simulink model "openloop"  (R2021b)
settings: Solver=ode15s  StartTime=0.0  StopTime=50  FixedStep=0.01  RelTol=1e-5  AbsTol=1e-8
values from neighbouring files (symbols this model uses):
  carb1 = 0    [olasm1init.m]
  carb2 = 0    [olasm1init.m]
  carb3 = 0    [olasm1init.m]
  carb4 = 0    [olasm1init.m]
  carb5 = 0    [olasm1init.m]
  DIM = [ area height ]    [olsettler1dinit.m]
  KLa1 = 0    [olasm1init.m]
  KLa2 = 0    [olasm1init.m]
  KLa3 = 240    [olasm1init.m]
  KLa4 = 240    [olasm1init.m]
  KLa5 = 84    [olasm1init.m]
  LAYER = [ feedlayer nooflayers ]    [olsettler1dinit.m]
  MODELTYPE = [ 0 ]    [olsettler1dinit.m]
  PAR1 = [ mu_H  K_S  K_OH  K_NO  b_H  mu_A  K_NH  K_OA  b_A  ny_g  k_a  k_h  K_X  ny_h  Y_H  Y_A  f_P  i_XB  i_XP X_I2TSS  X_S2TSS  X_BH2TSS  X_BA2TSS  X_P2TSS ]    [olasm1init.m]
  PAR2 = PAR1    [olasm1init.m]
  PAR3 = PAR1    [olasm1init.m]
  PAR4 = PAR1    [olasm1init.m]
  PAR5 = PAR1    [olasm1init.m]
  Qin0 = 18446    [olasm1init.m]    (also in statesetol.m)
  Qintr = 3*Qin0    (= 55338)    [olasm1init.m]    (also in statesetol.m)
  SETTLERINIT = [ TSS_1 TSS_2 TSS_3 TSS_4 TSS_5 TSS_6 TSS_7 TSS_8 TSS_9 TSS_10  SI_1 SI_2 SI_3 SI_4 SI_5 SI_6 SI_7 SI_8 SI_9 SI_10  SS_1 SS_2 SS_3 SS_4 SS_5 SS_6 SS_7 SS_8 SS_9 SS_10  SO_1 SO_2 SO_3 SO_4 SO_5 SO_6 SO_7 SO_8 SO_9 SO_10  SNO_1 SNO_2 SNO_3 SNO_4 SNO_5 SNO_6 SNO_7 SNO_8 SNO_9 SNO_10  SNH_1 SNH_2 SNH_3 SNH_4 SNH_5 SNH_6 SNH_7 SNH_8 SNH_9 SNH_10 SND_1 SND_2 SND_3 SND_4 SND_5 SND_6 SND_7 SND_8 SND_9 SND ...(+77 chars)    [olsettler1dinit.m]    (also in savestates.m; savestatesdyn.m; statesetol.m)
  SETTLERPAR = [ v0_max v0 r_h r_p f_ns X_t ]    [olsettler1dinit.m]
  SOSAT1 = 8    [olasm1init.m]
  SOSAT2 = SOSAT1    (= 8)    [olasm1init.m]
  SOSAT3 = SOSAT1    (= 8)    [olasm1init.m]
  SOSAT4 = SOSAT1    (= 8)    [olasm1init.m]
  SOSAT5 = SOSAT1    (= 8)    [olasm1init.m]
  T = 0.0002    [olasm1init.m]
  VOL1 = 1000    [olasm1init.m]
  VOL2 = VOL1    (= 1000)    [olasm1init.m]
  VOL3 = 1333    [olasm1init.m]
  VOL4 = VOL3    (= 1333)    [olasm1init.m]
  VOL5 = VOL3    (= 1333)    [olasm1init.m]
  XINIT1 = XINIT1.*(rand(1, 15)/2)    [olasm1init.m]    (also in savestates.m = [ S_I1  S_S1  X_I1  X_S1  X_BH1  X_BA1  X_P1  S_O1  S_NO1  S; savestatesdyn.m = [ S_I1  S_S1  X_I1  X_S1  X_BH1  X_BA1  X_P1  S_O1  S_NO1  S; statesetol.m = [ S_I1  S_S1  X_I1  X_S1  X_BH1  X_BA1  X_P1  S_O1  S_NO1  S)
  XINIT2 = XINIT2.*(rand(1, 15)/2)    [olasm1init.m]    (also in savestates.m = [ S_I2  S_S2  X_I2  X_S2  X_BH2  X_BA2  X_P2  S_O2  S_NO2  S; savestatesdyn.m = [ S_I2  S_S2  X_I2  X_S2  X_BH2  X_BA2  X_P2  S_O2  S_NO2  S; statesetol.m = [ S_I2  S_S2  X_I2  X_S2  X_BH2  X_BA2  X_P2  S_O2  S_NO2  S)
  XINIT3 = XINIT3.*(rand(1, 15)/2)    [olasm1init.m]    (also in savestates.m = [ S_I3  S_S3  X_I3  X_S3  X_BH3  X_BA3  X_P3  S_O3  S_NO3  S; savestatesdyn.m = [ S_I3  S_S3  X_I3  X_S3  X_BH3  X_BA3  X_P3  S_O3  S_NO3  S; statesetol.m = [ S_I3  S_S3  X_I3  X_S3  X_BH3  X_BA3  X_P3  S_O3  S_NO3  S)
  XINIT4 = XINIT4.*(rand(1, 15)/2)    [olasm1init.m]    (also in savestates.m = [ S_I4  S_S4  X_I4  X_S4  X_BH4  X_BA4  X_P4  S_O4  S_NO4  S; savestatesdyn.m = [ S_I4  S_S4  X_I4  X_S4  X_BH4  X_BA4  X_P4  S_O4  S_NO4  S; statesetol.m = [ S_I4  S_S4  X_I4  X_S4  X_BH4  X_BA4  X_P4  S_O4  S_NO4  S)
  XINIT5 = XINIT5.*(rand(1, 15)/2)    [olasm1init.m]    (also in savestates.m = [ S_I5  S_S5  X_I5  X_S5  X_BH5  X_BA5  X_P5  S_O5  S_NO5  S; savestatesdyn.m = [ S_I5  S_S5  X_I5  X_S5  X_BH5  X_BA5  X_P5  S_O5  S_NO5  S; statesetol.m = [ S_I5  S_S5  X_I5  X_S5  X_BH5  X_BA5  X_P5  S_O5  S_NO5  S)
  XINITDELAY = [ S_I_ASin  S_S_ASin  X_I_ASin  X_S_ASin  X_BH_ASin  X_BA_ASin  X_P_ASin  S_O_ASin  S_NO_ASin  S_NH_ASin  S_ND_ASin  X_ND_ASin  S_ALK_ASin TSS_ASin Q_ASin ]    [olasm1init.m]    (also in savestates.m; savestatesdyn.m; statesetol.m)
settings Model: Creator=ielulf  LastModifiedBy=Yalin
settings SolverCC: AutoScaleAbsTol=off  AlgebraicLoopSolver=TrustRegion
settings DataIOCC: LimitDataPoints=on  SaveFormat=Array  SignalLoggingSaveFormat=ModelDataLogs  SaveOutput=off  ReturnWorkspaceOutputs=off  TimeSaveName=t  SignalLoggingName=sigsOut  OutputOption=SpecifiedOutputTimes  OutputTimes=[0:1:50]
settings OptimizationCC: BlockReduction=off  BooleanDataType=off  InitFltsAndDblsToZero=on  LifeSpan=inf
settings DebuggingCC: SaveWithParameterizedLinksMsg=none  UnderspecifiedInitializationDetection=Classic  MergeDetectMultiDrivingBlocksExec=none  SignalResolutionControl=TryResolveAllWithWarning  InheritedTsInSrcMsg=none  MultiTaskDSMMsg=warning  MultiTaskCondExecSysMsg=none  FcnCallInpInsideContextMsg=warning  UnconnectedOutputMsg=none  SFUnexpectedBacktrackingDiag=warning  SFNoUnconditionalDefaultTransitionDiag=warning  SFExecutionAtInitializationDiag=none  SFMachineParentedDataDiag=warning  ArithmeticOperatorsInVariantConditions=warning
settings HardwareCC: ProdBitPerPointer=32  ProdBitPerSizeT=32  ProdBitPerPtrDiffT=32  ProdLargestAtomicFloat=None  ProdIntDivRoundTo=Undefined  ProdEndianess=Unspecified  ProdWordSize=32  ProdHWDeviceType=32-bit Generic  TargetUnknown=on
settings ModelReferenceCC: PropagateSignalLabelsOutOfModel=off
settings RTWCC: TemplateMakefile=grt_unix.tmf
settings CodeAppCC: StateflowObjectComments=on
settings GRTTargetCC: TargetFcnLib=ansi_tfl_tmw.mat  TargetLangStandard=C89/C90 (ANSI)  CombineOutputUpdateFcns=off  GRTInterface=on
settings ConfigComp: CovMetricSettings=dw  CovSaveCumulativeToWorkspaceVar=on  CovSaveSingleToWorkspaceVar=on

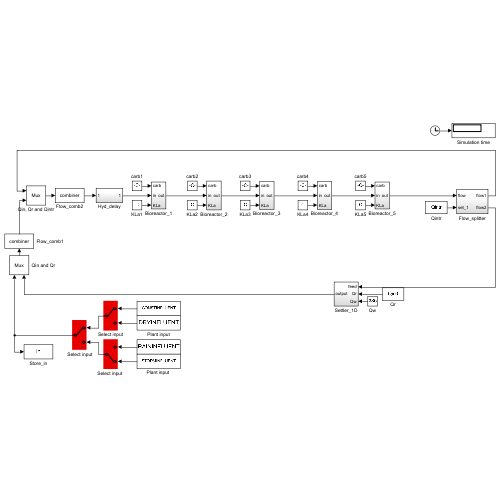
[thumbnail: Simulink's stored preview of the top-level diagram]
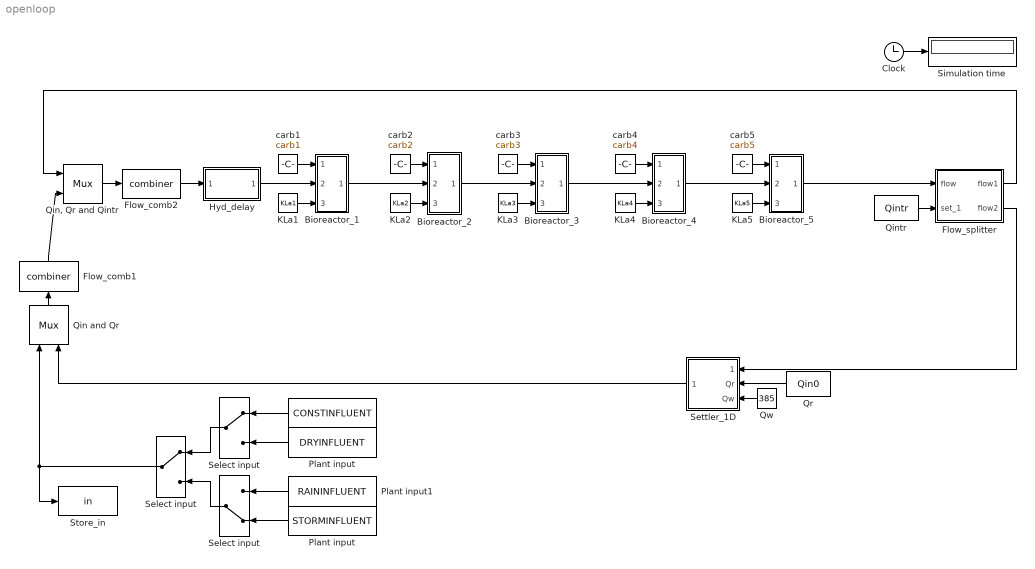
== system openloop ==
  " " : FromWorkspace  VariableName=CONSTINFLUENT  SampleTime=-1  ZeroCross=off  OutputAfterFinalValue=Holding final value
  " Select input" : ManualSwitch
  Bioreactor_1 : Subsystem
  Bioreactor_2 : Subsystem
  Bioreactor_3 : Subsystem
  Bioreactor_4 : Subsystem
  Bioreactor_5 : Subsystem
  Clock : Clock
  Flow_comb1 : S-Function  FunctionName=combiner  SFunctionDeploymentMode=off  EnableBusSupport=off
  Flow_comb2 : S-Function  FunctionName=combiner  SFunctionDeploymentMode=off  EnableBusSupport=off
  Flow_splitter : Subsystem
  Hyd_delay : Subsystem
  KLa1 : Constant  Value=KLa1
  KLa2 : Constant  Value=KLa2
  KLa3 : Constant  Value=KLa3
  KLa4 : Constant  Value=KLa4
  KLa5 : Constant  Value=KLa5
  Plant input : FromWorkspace  VariableName=DRYINFLUENT  SampleTime=-1  ZeroCross=off  OutputAfterFinalValue=Holding final value
  "Plant input " : FromWorkspace  VariableName=STORMINFLUENT  SampleTime=-1  ZeroCross=off  OutputAfterFinalValue=Holding final value
  Plant input1 : FromWorkspace  VariableName=RAININFLUENT  SampleTime=-1  ZeroCross=off  OutputAfterFinalValue=Holding final value
  Qin and Qr : Mux  Inputs=2
  "Qin, Qr and Qintr" : Mux  Inputs=2
  Qintr : Constant  Value=Qintr
  Qr : Constant  Value=Qin0
  Qw : Constant  Value=385
  Select input : ManualSwitch
  "Select input " : ManualSwitch  CurrentSetting=0
  Settler_1D : Subsystem
  Simulation time : Display
  Store_in : ToWorkspace  VariableName=in  SampleTime=-1
  carb1 : Constant  Value=carb1
  carb2 : Constant  Value=carb2
  carb3 : Constant  Value=carb3
  carb4 : Constant  Value=carb4
  carb5 : Constant  Value=carb5
  wires:
  Qin and Qr/1 -> Flow_comb1/1
  Flow_comb1/1 -> "Qin, Qr and Qintr"/2
  "Qin, Qr and Qintr"/1 -> Flow_comb2/1
  Flow_splitter/1(flow1) -> "Qin, Qr and Qintr"/1
  Settler_1D/1(output) -> Qin and Qr/2
  Qw/1 -> Settler_1D/3(Qw)
  Flow_splitter/2(flow2) -> Settler_1D/1(feed)
  Qintr/1 -> Flow_splitter/2(set_1)
  Qr/1 -> Settler_1D/2(Qr)
  Bioreactor_5/1(out) -> Flow_splitter/1(flow)
  Flow_comb2/1 -> Hyd_delay/1(Input)
  Clock/1 -> Simulation time/1
  Plant input/1 -> Select input/2
  " "/1 -> Select input/1
  Hyd_delay/1(Output) -> Bioreactor_1/2(in)
  carb1/1 -> Bioreactor_1/1(carb)
  KLa1/1 -> Bioreactor_1/3(KLa)
  Bioreactor_1/1(out) -> Bioreactor_2/2(in)
  KLa2/1 -> Bioreactor_2/3(KLa)
  carb2/1 -> Bioreactor_2/1(carb)
  Bioreactor_2/1(out) -> Bioreactor_3/2(in)
  KLa3/1 -> Bioreactor_3/3(KLa)
  carb3/1 -> Bioreactor_3/1(carb)
  Bioreactor_3/1(out) -> Bioreactor_4/2(in)
  KLa4/1 -> Bioreactor_4/3(KLa)
  carb4/1 -> Bioreactor_4/1(carb)
  Bioreactor_4/1(out) -> Bioreactor_5/2(in)
  KLa5/1 -> Bioreactor_5/3(KLa)
  carb5/1 -> Bioreactor_5/1(carb)
  Plant input1/1 -> "Select input "/1
  "Plant input "/1 -> "Select input "/2
  Select input/1 -> " Select input"/1
  "Select input "/1 -> " Select input"/2
  " Select input"/1 -> Qin and Qr/1, Store_in/1

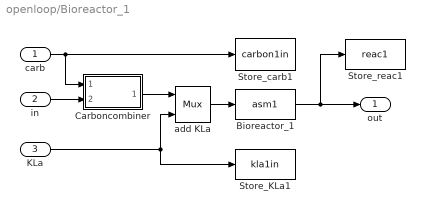
== system openloop/Bioreactor_1 ==
  carb : Inport
  in : Inport  Port=2
  KLa : Inport  Port=3
  Bioreactor_1 : S-Function  FunctionName=asm1  Parameters=XINIT1,PAR1,VOL1,SOSAT1  SFunctionDeploymentMode=off  EnableBusSupport=off
  Carboncombiner : Subsystem
  Store_KLa1 : ToWorkspace  VariableName=kla1in  SampleTime=-1
  Store_carb1 : ToWorkspace  VariableName=carbon1in  SampleTime=-1
  Store_reac1 : ToWorkspace  VariableName=reac1  SampleTime=-1
  add KLa : Mux  Inputs=2
  out : Outport
  wires:
  add KLa/1 -> Bioreactor_1/1
  Bioreactor_1/1 -> out/1, Store_reac1/1
  Carboncombiner/1(Output) -> add KLa/1
  carb/1 -> Store_carb1/1, Carboncombiner/1(C_flow)
  in/1 -> Carboncombiner/2(Input)
  KLa/1 -> add KLa/2, Store_KLa1/1

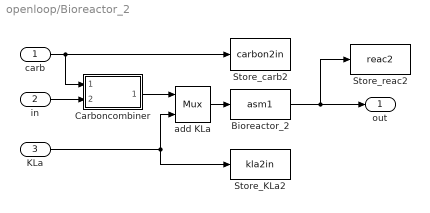
== system openloop/Bioreactor_2 ==
  carb : Inport
  in : Inport  Port=2
  KLa : Inport  Port=3
  Bioreactor_2 : S-Function  FunctionName=asm1  Parameters=XINIT2,PAR2,VOL2,SOSAT2  SFunctionDeploymentMode=off  EnableBusSupport=off
  Carboncombiner : Subsystem
  Store_KLa2 : ToWorkspace  VariableName=kla2in  SampleTime=-1
  Store_carb2 : ToWorkspace  VariableName=carbon2in  SampleTime=-1
  Store_reac2 : ToWorkspace  VariableName=reac2  SampleTime=-1
  add KLa : Mux  Inputs=2
  out : Outport
  wires:
  Bioreactor_2/1 -> out/1, Store_reac2/1
  add KLa/1 -> Bioreactor_2/1
  Carboncombiner/1(Output) -> add KLa/1
  carb/1 -> Carboncombiner/1(C_flow), Store_carb2/1
  in/1 -> Carboncombiner/2(Input)
  KLa/1 -> add KLa/2, Store_KLa2/1

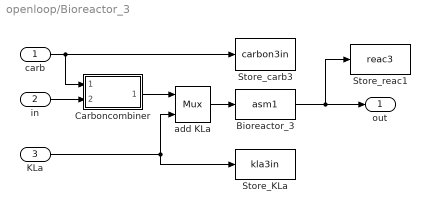
== system openloop/Bioreactor_3 ==
  carb : Inport
  in : Inport  Port=2
  KLa : Inport  Port=3
  Bioreactor_3 : S-Function  FunctionName=asm1  Parameters=XINIT3,PAR3,VOL3,SOSAT3  SFunctionDeploymentMode=off  EnableBusSupport=off
  Carboncombiner : Subsystem
  Store_KLa : ToWorkspace  VariableName=kla3in  SampleTime=-1
  Store_carb3 : ToWorkspace  VariableName=carbon3in  SampleTime=-1
  Store_reac1 : ToWorkspace  VariableName=reac3  SampleTime=-1
  add KLa : Mux  Inputs=2
  out : Outport
  wires:
  Bioreactor_3/1 -> out/1, Store_reac1/1
  add KLa/1 -> Bioreactor_3/1
  Carboncombiner/1(Output) -> add KLa/1
  carb/1 -> Carboncombiner/1(C_flow), Store_carb3/1
  in/1 -> Carboncombiner/2(Input)
  KLa/1 -> add KLa/2, Store_KLa/1

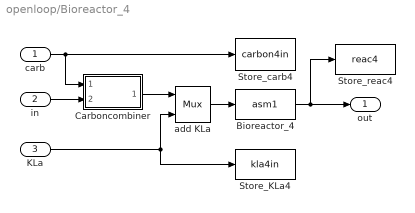
== system openloop/Bioreactor_4 ==
  carb : Inport
  in : Inport  Port=2
  KLa : Inport  Port=3
  Bioreactor_4 : S-Function  FunctionName=asm1  Parameters=XINIT4,PAR4,VOL4,SOSAT4  SFunctionDeploymentMode=off  EnableBusSupport=off
  Carboncombiner : Subsystem
  Store_KLa4 : ToWorkspace  VariableName=kla4in  SampleTime=-1
  Store_carb4 : ToWorkspace  VariableName=carbon4in  SampleTime=-1
  Store_reac4 : ToWorkspace  VariableName=reac4  SampleTime=-1
  add KLa : Mux  Inputs=2
  out : Outport
  wires:
  Bioreactor_4/1 -> out/1, Store_reac4/1
  add KLa/1 -> Bioreactor_4/1
  Carboncombiner/1(Output) -> add KLa/1
  carb/1 -> Carboncombiner/1(C_flow), Store_carb4/1
  in/1 -> Carboncombiner/2(Input)
  KLa/1 -> add KLa/2, Store_KLa4/1

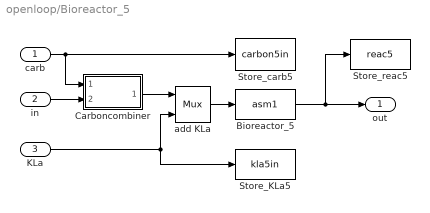
== system openloop/Bioreactor_5 ==
  carb : Inport
  in : Inport  Port=2
  KLa : Inport  Port=3
  Bioreactor_5 : S-Function  FunctionName=asm1  Parameters=XINIT5,PAR5,VOL5,SOSAT5  SFunctionDeploymentMode=off  EnableBusSupport=off
  Carboncombiner : Subsystem
  Store_KLa5 : ToWorkspace  VariableName=kla5in  SampleTime=-1
  Store_carb5 : ToWorkspace  VariableName=carbon5in  SampleTime=-1
  Store_reac5 : ToWorkspace  VariableName=reac5  SampleTime=-1
  add KLa : Mux  Inputs=2
  out : Outport
  wires:
  Bioreactor_5/1 -> out/1, Store_reac5/1
  add KLa/1 -> Bioreactor_5/1
  Carboncombiner/1(Output) -> add KLa/1
  carb/1 -> Carboncombiner/1(C_flow), Store_carb5/1
  in/1 -> Carboncombiner/2(Input)
  KLa/1 -> add KLa/2, Store_KLa5/1

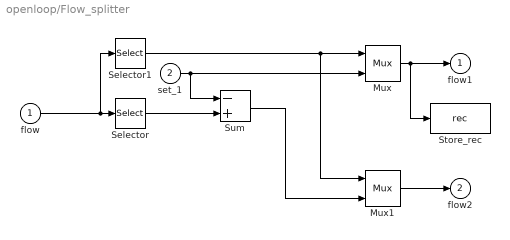
== system openloop/Flow_splitter ==
  flow : Inport
  set_1 : Inport  Port=2
  Mux : Mux  Inputs=2
  Mux1 : Mux  Inputs=2
  Selector : Selector  InputPortWidth=15  IndexOptions=Index vector (dialog)  Indices=[15]  OutputSizes=1
  Selector1 : Selector  InputPortWidth=15  IndexOptions=Index vector (dialog)  Indices=[1 2 3 4 5 6 7 8 9 10 11 12 13 14]  OutputSizes=1
  Store_rec : ToWorkspace  VariableName=rec  SampleTime=-1
  Sum : Sum  Inputs=-+  InputSameDT=on  SaturateOnIntegerOverflow=on  OutDataTypeStr=Inherit: Same as first input
  flow1 : Outport
  flow2 : Outport  Port=2
  wires:
  flow/1 -> Selector1/1, Selector/1
  Mux/1 -> flow1/1, Store_rec/1
  Mux1/1 -> flow2/1
  set_1/1 -> Mux/2, Sum/1
  Selector/1 -> Sum/2
  Sum/1 -> Mux1/2
  Selector1/1 -> Mux/1, Mux1/1

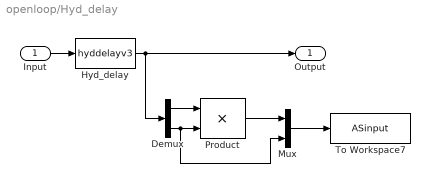
== system openloop/Hyd_delay ==
  Input : Inport
  Demux : Demux  Outputs=[14,1]
      settings: DisplayOption=none
  Hyd_delay : S-Function  FunctionName=hyddelayv3  Parameters=XINITDELAY,PAR1,T  SFunctionDeploymentMode=off  EnableBusSupport=off
  Mux : Mux  Inputs=2
  Product : Product  SaturateOnIntegerOverflow=on  OutDataTypeStr=Inherit: Same as first input
  To Workspace7 : ToWorkspace  VariableName=ASinput  SampleTime=-1
  Output : Outport
  wires:
  Input/1 -> Hyd_delay/1
  Hyd_delay/1 -> Output/1, Demux/1
  Demux/1 -> Product/1
  Demux/2 -> Product/2, Mux/2
  Product/1 -> Mux/1
  Mux/1 -> To Workspace7/1

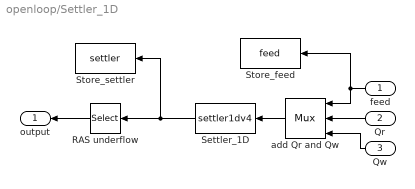
== system openloop/Settler_1D ==
  feed : Inport
  Qr : Inport  Port=2
  Qw : Inport  Port=3
  RAS underflow : Selector  InputPortWidth=113  IndexOptions=Index vector (dialog)  Indices=[1 2 3 4 5 6 7 8 9 10 11 12 13 14 15]  OutputSizes=1
  Settler_1D : S-Function  FunctionName=settler1dv4  Parameters=SETTLERINIT,SETTLERPAR,DIM,LAYER,MODELTYPE  SFunctionDeploymentMode=off  EnableBusSupport=off
  Store_feed : ToWorkspace  VariableName=feed  SampleTime=-1
  Store_settler : ToWorkspace  VariableName=settler  SampleTime=-1
  add Qr and Qw : Mux  Inputs=3
  output : Outport
  wires:
  add Qr and Qw/1 -> Settler_1D/1
  Qr/1 -> add Qr and Qw/2
  Qw/1 -> add Qr and Qw/3
  feed/1 -> add Qr and Qw/1, Store_feed/1
  RAS underflow/1 -> output/1
  Settler_1D/1 -> RAS underflow/1, Store_settler/1

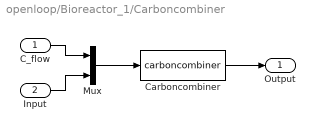
== system openloop/Bioreactor_1/Carboncombiner ==
  C_flow : Inport
  Input : Inport  Port=2
  Carboncombiner : S-Function  FunctionName=carboncombiner  Parameters=CARBONSOURCECONC  SFunctionDeploymentMode=off  EnableBusSupport=off
  Mux : Mux  Inputs=2
  Output : Outport
  wires:
  C_flow/1 -> Mux/1
  Mux/1 -> Carboncombiner/1
  Carboncombiner/1 -> Output/1
  Input/1 -> Mux/2

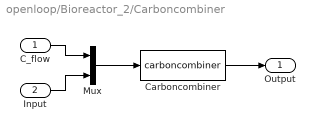
== system openloop/Bioreactor_2/Carboncombiner ==
  C_flow : Inport
  Input : Inport  Port=2
  Carboncombiner : S-Function  FunctionName=carboncombiner  Parameters=CARBONSOURCECONC  SFunctionDeploymentMode=off  EnableBusSupport=off
  Mux : Mux  Inputs=2
  Output : Outport
  wires:
  Input/1 -> Mux/2
  Carboncombiner/1 -> Output/1
  Mux/1 -> Carboncombiner/1
  C_flow/1 -> Mux/1

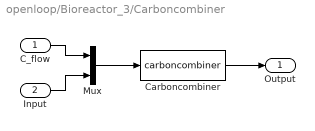
== system openloop/Bioreactor_3/Carboncombiner ==
  C_flow : Inport
  Input : Inport  Port=2
  Carboncombiner : S-Function  FunctionName=carboncombiner  Parameters=CARBONSOURCECONC  SFunctionDeploymentMode=off  EnableBusSupport=off
  Mux : Mux  Inputs=2
  Output : Outport
  wires:
  Input/1 -> Mux/2
  Carboncombiner/1 -> Output/1
  Mux/1 -> Carboncombiner/1
  C_flow/1 -> Mux/1

== system openloop/Bioreactor_4/Carboncombiner ==
  C_flow : Inport
  Input : Inport  Port=2
  Carboncombiner : S-Function  FunctionName=carboncombiner  Parameters=CARBONSOURCECONC  SFunctionDeploymentMode=off  EnableBusSupport=off
  Mux : Mux  Inputs=2
  Output : Outport
  wires:
  Input/1 -> Mux/2
  Carboncombiner/1 -> Output/1
  Mux/1 -> Carboncombiner/1
  C_flow/1 -> Mux/1

== system openloop/Bioreactor_5/Carboncombiner ==
  C_flow : Inport
  Input : Inport  Port=2
  Carboncombiner : S-Function  FunctionName=carboncombiner  Parameters=CARBONSOURCECONC  SFunctionDeploymentMode=off  EnableBusSupport=off
  Mux : Mux  Inputs=2
  Output : Outport
  wires:
  Input/1 -> Mux/2
  Carboncombiner/1 -> Output/1
  Mux/1 -> Carboncombiner/1
  C_flow/1 -> Mux/1
